simulink model "Izhikevich_Neuron_Model"  (R2017b)
settings: Solver=VariableStepAuto  StartTime=0.0  StopTime=500  MaxStep=0.1  MinStep=0.01  RelTol=1e-3
settings Model: Creator=Lenovo  LastModifiedBy=Lenovo

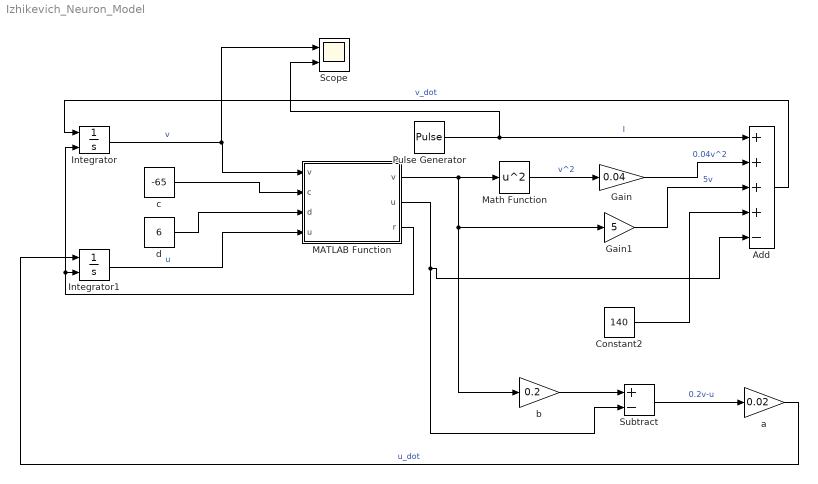
== system Izhikevich_Neuron_Model ==
  Add : Sum  Inputs=++++-
  Constant2 : Constant  Value=140
  Gain : Gain  Gain=0.04
  Gain1 : Gain  Gain=5
  Integrator : Integrator  ExternalReset=rising  InitialCondition=-65  LimitOutput=on  UpperSaturationLimit=30
  Integrator1 : Integrator  ExternalReset=rising  InitialCondition=6
  MATLAB Function : MATLAB Function  TreatAsAtomicUnit=on
  Math Function : Math  Operator=square  SaturateOnIntegerOverflow=on
  Pulse Generator : DiscretePulseGenerator  PulseType=Time based  Amplitude=0  Period=250  PulseWidth=50  PhaseDelay=60
  Scope : Scope  NumInputPorts=2
  Subtract : Sum  Inputs=+-
  a : Gain  Gain=0.02
  b : Gain  Gain=0.2
  c : Constant  Value=-65
  d : Constant  Value=6
  wires:
  Add/1 -> Integrator/1  "v_dot"
  Integrator/1 -> Scope/1, MATLAB Function/1("v ")  "v"
  Integrator1/1 -> MATLAB Function/4("u ")  "u"
  a/1 -> Integrator1/1  "u_dot"
  c/1 -> MATLAB Function/2(c)
  d/1 -> MATLAB Function/3(d)
  Pulse Generator/1 -> Scope/2, Add/1  "I"
  MATLAB Function/1(v) -> Gain1/1, b/1, Math Function/1
  Math Function/1 -> Gain/1  "v^2"
  Constant2/1 -> Add/4
  MATLAB Function/3(r) -> Integrator/2, Integrator1/2
  b/1 -> Subtract/1
  MATLAB Function/2(u) -> Add/5, Subtract/2
  Subtract/1 -> a/1  "0.2v-u"
  Gain/1 -> Add/2  "0.04v^2"
  Gain1/1 -> Add/3  "5v"

== matlab function Izhikevich_Neuron_Model/MATLAB Function ==
  data: v input; c input; d input; u input; v output; u output; r output
function [v, u, r] = repolarization(v, c, d, u)

if v >= 30
    v = c;
    u = c + d;
    r = 1;
else
    r = 0;
end
